simulink model "TrafficLightComposer"  (R2022a)
settings: Solver=FixedStepDiscrete  StartTime=0.0  StopTime=1000  FixedStep=1  MaxStep=1  RelTol=1e-3
settings Model: DataDictionary=TrafficLightComposer.sldd  NumberOfSteps=5  SnapshotBufferSize=100  PacingRate=5  Creator=Amin  LastModifiedBy=Amin
settings SolverCC: ConsecutiveZCsStepRelTol=100*128*eps

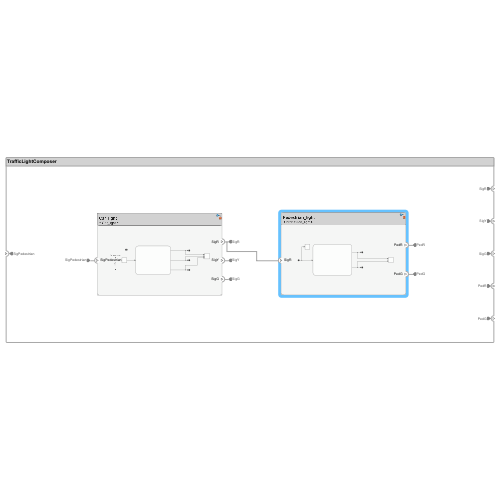
[thumbnail: Simulink's stored preview of the top-level diagram]
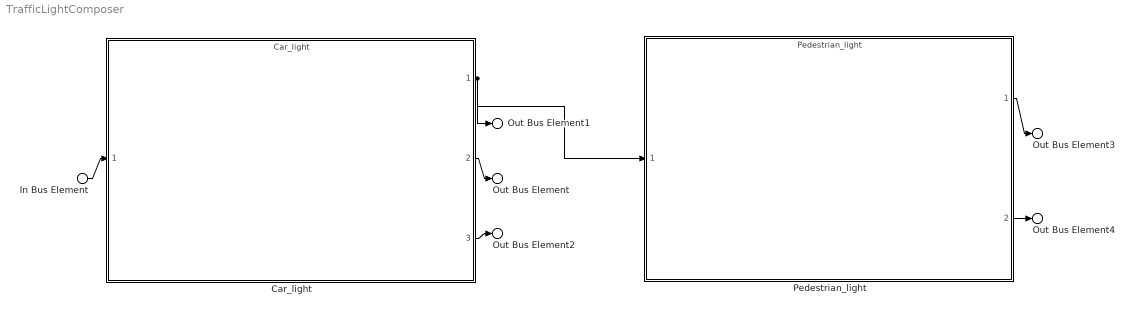
== system TrafficLightComposer ==
  In Bus Element : Inport  PortName=SigPedestrian
  Car_light : ModelReference  ModelNameDialog=Car_light  SimulationMode=Normal  ModelReferenceVersion=1.22
      settings: PortSchema="{\"entries\":[{\"content\":{\"headerSize\":38,\"margin\":15,\"minimumSpacing\":25,\"sides\":[{\"content\":{\"connectorIds\":[\"In1\"]},\"type\":\"ConnectorPlacement.EquallySpacedRectSide\",\"uuid\":\"4fc7b3d1-356b-453a-bb43-7052b9275e66\"},{\"content\":{\"connectorIds\":[\"Out1\",\"Out2\",\"Out3\"],\"side\":\"RIGHT\"},\"type\":\"ConnectorPlacement.EquallySpacedRectSide\",\"uuid\":\"a2d7123c-8d9a-4168-9f8f-97b3cad3aa67\"},{\"content\":{\"connectorIds\":[],\"side\":\"TOP\"},\"type\":\"ConnectorPlacement.EquallySpacedRectSide\",\"uuid\":\"e1226b7a-6cf9-4837-8d00-8a6da23e4d69\"}]},\"type\":\"ConnectorPlacement.EquallySpacedConnector\",\"uuid\":\"b7566362-4911-4718-ba1c-12724fb08052\"}],\"packageUris\":[\"http://schema.mathworks.com/mf0/Connector/R2020b\"],\"version\":\"1.0\"}"
  Pedestrian_light : ModelReference  ModelNameDialog=Pedestrian_light  SimulationMode=Normal  ModelReferenceVersion=1.12
      settings: PortSchema="{\"entries\":[{\"content\":{\"headerSize\":38,\"margin\":15,\"minimumSpacing\":25,\"sides\":[{\"content\":{\"connectorIds\":[\"In1\"]},\"type\":\"ConnectorPlacement.EquallySpacedRectSide\",\"uuid\":\"1768163e-7bc3-4b21-b0d1-16e00818ee39\"},{\"content\":{\"connectorIds\":[\"Out1\",\"Out2\"],\"side\":\"RIGHT\"},\"type\":\"ConnectorPlacement.EquallySpacedRectSide\",\"uuid\":\"73701803-853b-40ad-ac69-982147da3f18\"},{\"content\":{\"connectorIds\":[],\"side\":\"TOP\"},\"type\":\"ConnectorPlacement.EquallySpacedRectSide\",\"uuid\":\"b798a976-d374-49d1-9a5c-ffade60bf3f9\"}]},\"type\":\"ConnectorPlacement.EquallySpacedConnector\",\"uuid\":\"751ea083-3651-40de-9df1-9b7db637cc15\"}],\"packageUris\":[\"http://schema.mathworks.com/mf0/Connector/R2020b\"],\"version\":\"1.0\"}"
  Out Bus Element1 : Outport  PortName=SigR
  Out Bus Element : Outport  Port=2  PortName=SigY
  Out Bus Element2 : Outport  Port=3  PortName=SigG
  Out Bus Element3 : Outport  Port=4  PortName=PedR
  Out Bus Element4 : Outport  Port=5  PortName=PedG
  wires:
  In Bus Element/1 -> Car_light/1
  Car_light/1 -> Out Bus Element1/1, Pedestrian_light/1
  Car_light/2 -> Out Bus Element/1
  Pedestrian_light/1 -> Out Bus Element3/1
  Car_light/3 -> Out Bus Element2/1
  Pedestrian_light/2 -> Out Bus Element4/1
